simulink model "WiberSystemMultiModes"  (R2022b)
settings: Solver=VariableStepAuto  StartTime=0.0  StopTime=inf  MaxStep=1e-3  RelTol=1e-3
libraries: spsSawtoothGeneratorLib x1
(part 2 of 2)

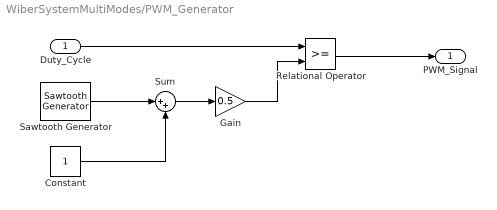
== system WiberSystemMultiModes/PWM_Generator ==
  Duty_Cycle : Inport
  Constant : Constant
  Gain : Gain  Gain=0.5
  Relational Operator : RelationalOperator  OutDataTypeStr=boolean  RndMeth=Simplest  InputSameDT=off
  Sawtooth Generator : spsSawtoothGeneratorLib/Sawtooth Generator  Freq=0.1  Phase=0  Ts=0
  Sum : Sum  Inputs=|++
  PWM_Signal : Outport
  wires:
  Relational Operator/1 -> PWM_Signal/1
  Sawtooth Generator/1 -> Sum/1
  Constant/1 -> Sum/2
  Gain/1 -> Relational Operator/2
  Sum/1 -> Gain/1
  Duty_Cycle/1 -> Relational Operator/1

== stateflow chart WiberSystemMultiModes/Wiber_System_Logic ==
  state OFF
    entry: Duty_Cycle = 0;
  state AUTO
    entry: Duty_Cycle = 0.8*Rain_Intinsity;
    % 0.8 is a random choice
  state HIGH
    entry: Duty_Cycle = 0.7;
  state LOW
    entry: Duty_Cycle = 0.4;
  AUTO -> HIGH [order 3] : [Mode == 3]
  (default) -> OFF
  AUTO -> OFF [order 2] : [Mode == 0]
  OFF -> HIGH [order 1] : [Mode == 3]
  OFF -> AUTO [order 2] : [Mode == 1]
  HIGH -> OFF [order 1] : [Mode == 0]
  LOW -> OFF [order 1] : [Mode == 0]
  OFF -> LOW [order 3] : [Mode == 2]
  HIGH -> AUTO [order 3] : [Mode == 1]
  HIGH -> LOW [order 2] : [Mode == 2]
  LOW -> HIGH [order 3] : [Mode == 3]
  AUTO -> LOW [order 1] : [Mode == 2]
  LOW -> AUTO [order 2] : [Mode == 1]
  data: Mode input; Duty_Cycle output; Rain_Intinsity input
